simulink model "ifo_ut"  (Simulink 8.1)
settings: Solver=FixedStepDiscrete  StartTime=0.0  StopTime=10.0  FixedStep=0.005  RelTol=1e-3
PostLoadFcn:
  | , if any(exist('dsrtsu_mdlpostloadfcn', 'file') == [2, 3, 6]), try dsrtsu_mdlpostloadfcn('Execute', bdroot); catch fprintf('Error in PostLoadFcn (dsrtsu_mdlpostloadfcn) for model "%s":\n %s\n', bdroot, lasterr); end, end,
undefined symbols (not defined in the file or in its folder): VACC_ACCActing_flg, VACC_ACCOverride_flg, VACC_ACCRawTorqueReq_Nm, VACC_ACCSystemState_enum, VACC_DesiredDistance_m, VACC_StandstillClearance_m, VAEB_AEBActing_flg, VAEB_AEBSystemState_enum, VDHP_DisableACC_flg, VDHP_DisableADASFun_flg, VIFO_ACCCancelReq_flg, VIFO_ACCDist_flg, VIFO_ACCResSpdInc_flg, VIFO_ACCSetSpdDec_flg, VIFO_ACCTargetVehAssigned_flg, VIFO_ACCTargetVehRelSpeedX_mps, VIFO_ACCVehClearance_m, VIFO_DriverOvertakeReq_flg, VIFO_DriverSafetyStatusOk_flg, VIFO_DriverTurnSignalOn_flg, VIFO_VehicleStatusOk_flg, VPER_CameraStatus_enum, VPER_FusionStatus_enum, VPER_RadarStatus_enum
libraries: siltestlib x32, ifo x1
settings Model: DSRTSU_INTERNAL_RTI_VER=450  DSRTSU_INTERNAL_RTI_TYPE=rti1401  RTICANMMDATA=struct('GeneralSetupData',struct('modelroot','D:\ELN150201_TAIWAN\trunk\AdasDragon\software\sw_development\arch\app\ifo','generalsettings',struct('filesettings',struct('destfolder',struct('Name','RTICANMM_FILES','Check',1),'buildfolder',struct('Name','.','Check',1),'AbsDestfolder',struct('Name','D:\ELN150201_TAIWAN\trunk\AdasDragon\software\sw_development\arch\app\ifo\RTICANMM_FILES'),'AbsBuildfolder',struct('Name','D:\ELN150201_TAIWAN\trunk\AdasDragon\software\sw_development\arch\app\ifo'))),'options',struct('addpaths',1,'rmpaths',1,'addtrcexclusion',logical(1),'cannavigator',struct('checkmonitoring',0),'show_usrtrc',0,'use_usrtrc',0),'advanced',struct('options',[1 1 1 1 1 1 1 1 1 1 1 1 1 1 1 1 1 1 1 1 1 1 1 1 1 1 1 1 1 1 1 1 1 1 1 1 1 1 1 1 1 1 1 1 1 1 1 1 1 1 1 1 1 1 1 1 1 1 1 1 1 1 1 1 1 1 1 1 1 1 1 1 1 1 1 1 1 1 1 1 1 1 1 1 1 1 1 1 1 1 1 1 1 1 1 1 1 1 1 1]),'MPSetup',{{}},'modelname','ifo_ut','block','ifo_ut'))  DSRTSU_INTERNAL_RTIFPGA=40  Creator=xsellart  LastModifiedBy=AT015555
settings DataIOCC: SignalLoggingSaveFormat=Dataset
settings OptimizationCC: ExpressionDepthLimit=128
settings DebuggingCC: FcnCallInpInsideContextMsg=EnableAllAsError
settings HardwareCC: ProdIntDivRoundTo=Zero  ProdEndianess=BigEndian  ProdHWDeviceType=Generic->Custom  TargetIntDivRoundTo=Zero  TargetEndianess=BigEndian  TargetHWDeviceType=Generic->Custom
settings RTWCC: SystemTargetFile=rti1401.tlc  MakeCommand=make_rti  TemplateMakefile=rti1401.tmf  Description=dSPACE DS1401 Hardware Platform  ProcessScript=rti1401_make_rtw_hook
settings STFCustomTargetCC: CodeReplacementLibrary=ANSI_C  ParMdlRefBuildCompliant=on  GeneratePreprocessorConditionals=Disable all  SystemTargetFile=rti1401.tlc
settings GRTTargetCC: CompOptLevelCompliant=off  ConcurrentExecutionCompliant=off  MatFileLogging=off  ExtModeMexFile=noextcomm
settings CustomProperty: DataType=RTWOptions_EnumType_C__Program Files (x86)_dSPACE RCPHIL 2014-B_MATLAB_RTI_RTI1401_TLC_rti1401_1InitialSimState  Value=RUN
settings EnumStrPairs: String=RUN

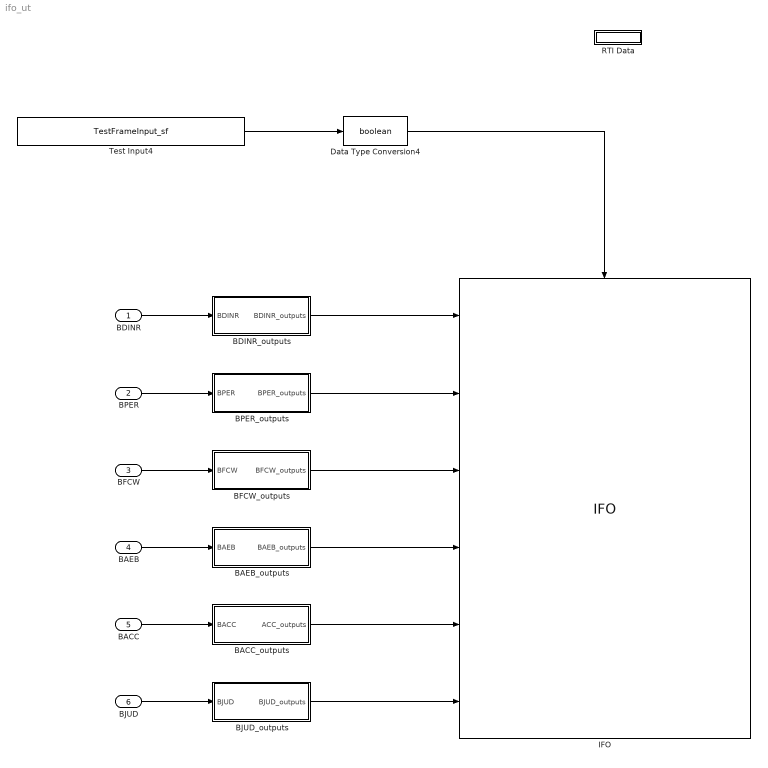
== system ifo_ut ==
  BDINR : Inport  OutDataTypeStr=Bus: BDINR_outputs
  BPER : Inport  Port=2  OutDataTypeStr=Bus: BPER_outputs
  BFCW : Inport  Port=3  OutDataTypeStr=Bus: BFCW_outputs
  BAEB : Inport  Port=4  OutDataTypeStr=Bus: BAEB_outputs
  BACC : Inport  Port=5  OutDataTypeStr=Bus: BACC_outputs
  BJUD : Inport  Port=6  OutDataTypeStr=Bus: BJUD_outputs
  BACC_outputs : Subsystem
  BAEB_outputs : Subsystem
  BDINR_outputs : Subsystem
  BFCW_outputs : Subsystem
  BJUD_outputs : Subsystem
  BPER_outputs : Subsystem
  Data Type Conversion4 : DataTypeConversion  OutDataTypeStr=boolean
  IFO : ifo/IFO
  RTI Data : Subsystem  Tag=struct('RTIDataServer',struct('RTIDataServerVs','2','RTIModelDescription','struct(''main'',''ifo_ut'',''sub'','''',''isMp'',0)'))  LoadFcn="if exist('rtidc'), try,  rtidc('DataHostBlockClbLoad', gcbh); catch, disp(['Warning: ''LoadFcn'' for RTI Data block failed: ' lasterr]); end, end,"  mask(RTI_DATA_HOST){}
      mask help:
      | RTI Data Block.
      | This block is used by RTI to store internal model-dependent data.
      | Please keep this block on the root level of the model. Deleting this block will result in data loss.
      |
      | NEVER DELETE OR COPY THIS BLOCK!
      settings: CopyFcn="if exist('rtidc'), try,  rtidc('DataHostBlockClbCopy', gcbh); catch, disp(['Warning: ''CopyFcn'' for RTI Data block failed: ' lasterr]); end, end,"  DeleteFcn="if exist('rtidc'), try,  rtidc('DataHostBlockClbDelete', gcbh); catch, disp(['Warning: ''DeleteFcn'' for RTI Data block failed: ' lasterr]); end, end,"  ModelCloseFcn="if exist('rtidc'), try,  rtidc('DataHostBlockClbModelClose', gcbh); catch, disp(['Warning: ''ModelCloseFcn'' for RTI Data block failed: ' lasterr]); end, end,"  PreSaveFcn="if exist('rtidc'), try,  rtidc('DataHostBlockClbPreSave', gcbh); catch, disp(['Warning: ''PreSaveFcn'' for RTI Data block failed: ' lasterr]); end, end,"  PostSaveFcn="if exist('rtidc'), try,  rtidc('DataHostBlockClbPostSave', gcbh); catch, disp(['Warning: ''PostSaveFcn'' for RTI Data block failed: ' lasterr]); end, end,"  NameChangeFcn="if exist('rtidc'), try,  rtidc('DataHostBlockClbNameChange', gcbh); catch, disp(['Warning: ''NameChangeFcn'' for RTI Data block failed: ' lasterr]); end, end,"
      mask Help:
      | RTI Data Block.
      | This block is used by RTI to store internal model-dependent data.
      | Please keep this block on the root level of the model. Deleting this block will result in data loss.
      | 
      | NEVER DELETE OR COPY THIS BLOCK!
      mask Display:
      | text(0.5, 0.5, 'RTI Data', 'HorizontalAlignment', 'center');
      | plot([1 0]);
  Test Input4 : S-Function  FunctionName=TestFrameInput_sf  Parameters=varname,sampletime  EnableBusSupport=off  mask(Test Input){varname=Scheduler_Trigger, sampletime=-1}
      mask prompts: varname "Name:"; sampletime "Sample Time:"
      mask help: Outputs the value of a Test Input variable from an Excel spreadsheet when used with the runsiltest script. Otherwise outputs 0.
      mask Display: fprintf('Test Input:\n%s',varname);
  wires:
  BDINR/1 -> BDINR_outputs/1(BDINR)
  BPER/1 -> BPER_outputs/1(BPER)
  BFCW/1 -> BFCW_outputs/1(BFCW)
  BJUD/1 -> BJUD_outputs/1(BJUD)
  BAEB/1 -> BAEB_outputs/1(BAEB)
  BACC/1 -> BACC_outputs/1(BACC)
  BFCW_outputs/1(BFCW_outputs) -> IFO/3
  BJUD_outputs/1(BJUD_outputs) -> IFO/6
  BACC_outputs/1(ACC_outputs) -> IFO/5
  BPER_outputs/1(BPER_outputs) -> IFO/2
  BDINR_outputs/1(BDINR_outputs) -> IFO/1
  BAEB_outputs/1(BAEB_outputs) -> IFO/4
  Test Input4/1 -> Data Type Conversion4/1
  Data Type Conversion4/1 -> IFO/Trigger

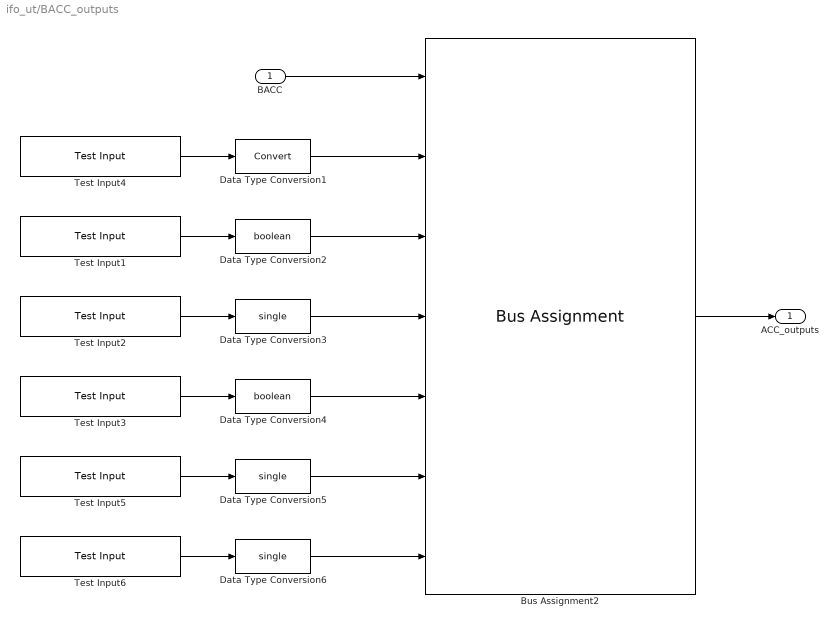
== system ifo_ut/BACC_outputs ==
  BACC : Inport  OutDataTypeStr=Bus: BACC_outputs
  Bus Assignment2 : BusAssignment  AssignedSignals=VACC_ACCSystemState_enum,VACC_ACCActing_flg,VACC_ACCRawTorqueReq_Nm,VACC_ACCOverride_flg,VACC_DesiredDistance_m,VACC_StandstillClearance_m
  Data Type Conversion1 : DataTypeConversion
  Data Type Conversion2 : DataTypeConversion  OutDataTypeStr=boolean
  Data Type Conversion3 : DataTypeConversion  OutDataTypeStr=single
  Data Type Conversion4 : DataTypeConversion  OutDataTypeStr=boolean
  Data Type Conversion5 : DataTypeConversion  OutDataTypeStr=single
  Data Type Conversion6 : DataTypeConversion  OutDataTypeStr=single
  Test Input1 : siltestlib/Test Input  varname=VACC_ACCActing_flg  sampletime=-1
  Test Input2 : siltestlib/Test Input  varname=VACC_ACCRawTorqueReq_Nm  sampletime=-1
  Test Input3 : siltestlib/Test Input  varname=VACC_ACCOverride_flg  sampletime=-1
  Test Input4 : siltestlib/Test Input  varname=VACC_ACCSystemState_enum  sampletime=-1
  Test Input5 : siltestlib/Test Input  varname=VACC_DesiredDistance_m  sampletime=-1
  Test Input6 : siltestlib/Test Input  varname=VACC_StandstillClearance_m  sampletime=-1
  ACC_outputs : Outport  OutDataTypeStr=Bus: BAEB_outputs
  wires:
  Test Input4/1 -> Data Type Conversion1/1
  Bus Assignment2/1 -> ACC_outputs/1
  BACC/1 -> Bus Assignment2/1
  Test Input1/1 -> Data Type Conversion2/1
  Test Input2/1 -> Data Type Conversion3/1
  Test Input3/1 -> Data Type Conversion4/1
  Test Input5/1 -> Data Type Conversion5/1
  Test Input6/1 -> Data Type Conversion6/1
  Data Type Conversion1/1 -> Bus Assignment2/2
  Data Type Conversion6/1 -> Bus Assignment2/7
  Data Type Conversion2/1 -> Bus Assignment2/3
  Data Type Conversion5/1 -> Bus Assignment2/6
  Data Type Conversion4/1 -> Bus Assignment2/5
  Data Type Conversion3/1 -> Bus Assignment2/4

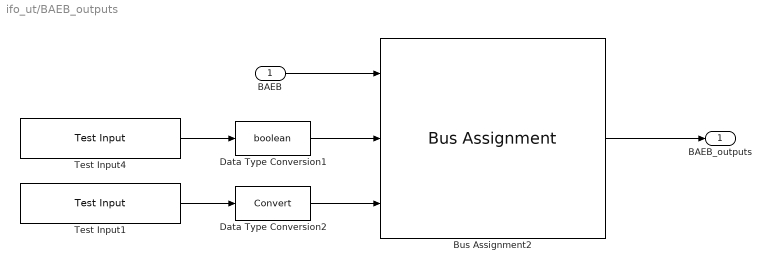
== system ifo_ut/BAEB_outputs ==
  BAEB : Inport  OutDataTypeStr=Bus: BAEB_outputs
  Bus Assignment2 : BusAssignment  AssignedSignals=VAEB_AEBActing_flg,VAEB_AEBSystemState_enum
  Data Type Conversion1 : DataTypeConversion  OutDataTypeStr=boolean
  Data Type Conversion2 : DataTypeConversion
  Test Input1 : siltestlib/Test Input  varname=VAEB_AEBSystemState_enum  sampletime=-1
  Test Input4 : siltestlib/Test Input  varname=VAEB_AEBActing_flg  sampletime=-1
  BAEB_outputs : Outport  OutDataTypeStr=Bus: BAEB_outputs
  wires:
  BAEB/1 -> Bus Assignment2/1
  Bus Assignment2/1 -> BAEB_outputs/1
  Test Input4/1 -> Data Type Conversion1/1
  Data Type Conversion1/1 -> Bus Assignment2/2
  Test Input1/1 -> Data Type Conversion2/1
  Data Type Conversion2/1 -> Bus Assignment2/3

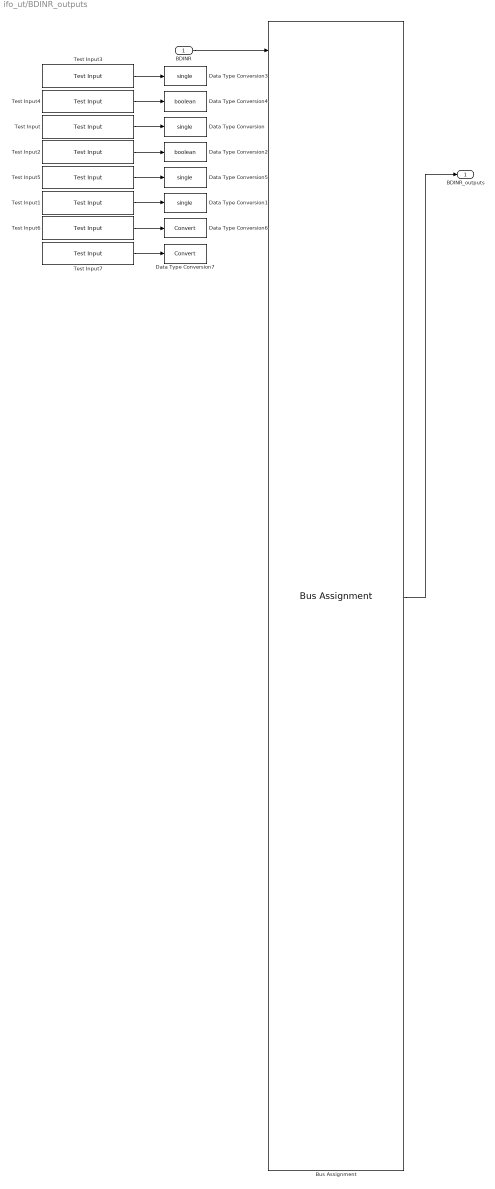
== system ifo_ut/BDINR_outputs ==
  BDINR : Inport  OutDataTypeStr=Bus: BDINR_outputs
  Bus Assignment : BusAssignment  AssignedSignals=VDINR_VehSpd_mps,VDINR_YawRate_degps,VDINR_SeatBeltNOTFasten_flg,VDINR_VehCrashed_flg,VDINR_TCSActive_flg,VDINR_VehSpdValid_flg,VDINR_LongAccelValid_flg,VDINR_LatAccelValid_flg,VDINR_YawRateValid_flg,VDINR_SteerAngleValid_flg,VDINR_SteerSpeedValid_flg,VDINR_HWAccelPedalPosnValid_flg,VDINR_DriverBrakPedalOnValid_flg,VDINR_NowGearPosnValid_flg,VDINR_ESCFault_flg,VDINR_ABSFault_flg,VDINR_EMSOpState_enum,VDINR_EPASMILReq_flg,VDINR_TCMFaultStatus_enum,VDINR_DriverDoorOpen_flg,VDINR_PassengerDoorOpen_flg,VDINR_LRDoorOpen_flg,VDINR_RRDoorOpen_flg,VDINR_SteerSpeed_degps,VDINR_SteerAngle_deg,VDINR_HWAccelPedalPosn_pct,VDINR_ParkBrakeBindSta_enum,VDINR_MCPressure_bar,VDINR_DriverBrakPedalOn_flg,VDINR_NowGearPosn_enum,VDINR_ACCOnVCU_flg,VDINR_TurnSignalSwL_flg,VDINR_TurnSignalSwR_flg,VDINR_LongAccel_G,VDINR_ACCSetSpdDecH_flg,VDINR_ACCSpdDecH_flg,VDINR_ACCResSpdIncH_flg,VDINR_ACCSpdIncH_flg,VDINR_ACCSetSpdDecVCU_flg,VDINR_ACCResSpdIncVCU_flg,VDINR_ACCDistVCU_flg,VDINR_ACCTimeGapDecH_flg,VDINR_ACCOnH_flg
  Data Type Conversion{,1,3,5} (4 alike) : DataTypeConversion  OutDataTypeStr=single
  Data Type Conversion2 : DataTypeConversion  OutDataTypeStr=boolean
  Data Type Conversion4 : DataTypeConversion  OutDataTypeStr=boolean
  Data Type Conversion6 : DataTypeConversion
  Data Type Conversion7 : DataTypeConversion
  Test Input : siltestlib/Test Input  varname=VDINR_VehSpd_kph  sampletime=-1
  Test Input1 : siltestlib/Test Input  varname=VDINR_CurDriverTqReq_Nm  sampletime=-1
  Test Input2 : siltestlib/Test Input  varname=VDINR_DriverBrakPedalOn_flg  sampletime=-1
  Test Input3 : siltestlib/Test Input  varname=VDINR_VehSpd_mps  sampletime=-1
  Test Input4 : siltestlib/Test Input  varname=VDINR_HMICANValid_flg  sampletime=-1
  Test Input5 : siltestlib/Test Input  varname=VDINR_HWAccelPedalPosn_pct  sampletime=-1
  Test Input6 : siltestlib/Test Input  varname=VDINR_NowGearPosn_enum  sampletime=-1
  Test Input7 : siltestlib/Test Input  varname=VDINR_ParkBrakeBindSta_enum  sampletime=-1
  BDINR_outputs : Outport  OutDataTypeStr=Bus: BDINR_outputs
  wires:
  Bus Assignment/1 -> BDINR_outputs/1
  BDINR/1 -> Bus Assignment/1
  Test Input/1 -> Data Type Conversion/1
  Test Input1/1 -> Data Type Conversion1/1
  Test Input2/1 -> Data Type Conversion2/1
  Test Input3/1 -> Data Type Conversion3/1
  Test Input4/1 -> Data Type Conversion4/1
  Test Input5/1 -> Data Type Conversion5/1
  Test Input6/1 -> Data Type Conversion6/1
  Test Input7/1 -> Data Type Conversion7/1

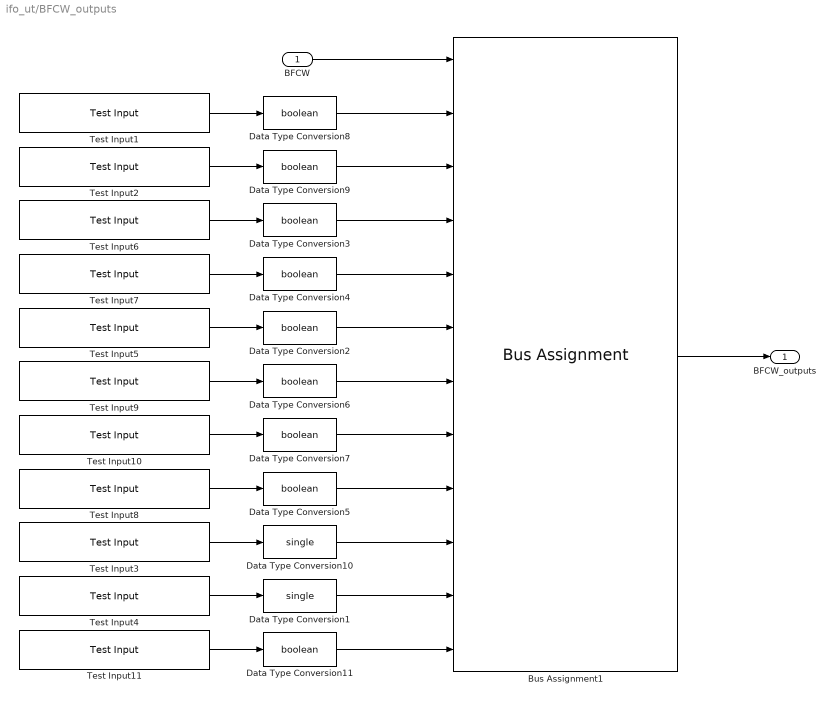
== system ifo_ut/BFCW_outputs ==
  BFCW : Inport  OutDataTypeStr=Bus: BFCW_outputs
  Bus Assignment1 : BusAssignment  AssignedSignals=VIFO_ACCSetSpdDec_flg,VIFO_ACCResSpdInc_flg,VIFO_ACCDist_flg,VIFO_ACCCancelReq_flg,VIFO_DriverOvertakeReq_flg,VIFO_VehicleStatusOk_flg,VIFO_DriverSafetyStatusOk_flg,VIFO_ACCTargetVehAssigned_flg,VIFO_ACCTargetVehRelSpeedX_mps,VIFO_ACCVehClearance_m,VIFO_DriverTurnSignalOn_flg
  Data Type Conversion1 : DataTypeConversion  OutDataTypeStr=single
  Data Type Conversion10 : DataTypeConversion  OutDataTypeStr=single
  Data Type Conversion{2..9,11} (9 alike) : DataTypeConversion  OutDataTypeStr=boolean
  Test Input1 : siltestlib/Test Input  varname=VIFO_ACCSetSpdDec_flg  sampletime=-1
  Test Input10 : siltestlib/Test Input  varname=VIFO_DriverSafetyStatusOk_flg  sampletime=-1
  Test Input11 : siltestlib/Test Input  varname=VIFO_DriverTurnSignalOn_flg  sampletime=-1
  Test Input2 : siltestlib/Test Input  varname=VIFO_ACCResSpdInc_flg  sampletime=-1
  Test Input3 : siltestlib/Test Input  varname=VIFO_ACCTargetVehRelSpeedX_mps  sampletime=-1
  Test Input4 : siltestlib/Test Input  varname=VIFO_ACCVehClearance_m  sampletime=-1
  Test Input5 : siltestlib/Test Input  varname=VIFO_DriverOvertakeReq_flg  sampletime=-1
  Test Input6 : siltestlib/Test Input  varname=VIFO_ACCDist_flg  sampletime=-1
  Test Input7 : siltestlib/Test Input  varname=VIFO_ACCCancelReq_flg  sampletime=-1
  Test Input8 : siltestlib/Test Input  varname=VIFO_ACCTargetVehAssigned_flg  sampletime=-1
  Test Input9 : siltestlib/Test Input  varname=VIFO_VehicleStatusOk_flg  sampletime=-1
  BFCW_outputs : Outport  OutDataTypeStr=Bus: BFCW_outputs
  wires:
  BFCW/1 -> Bus Assignment1/1
  Bus Assignment1/1 -> BFCW_outputs/1
  Test Input1/1 -> Data Type Conversion8/1
  Data Type Conversion8/1 -> Bus Assignment1/2
  Test Input2/1 -> Data Type Conversion9/1
  Data Type Conversion9/1 -> Bus Assignment1/3
  Test Input3/1 -> Data Type Conversion10/1
  Data Type Conversion3/1 -> Bus Assignment1/4
  Test Input4/1 -> Data Type Conversion1/1
  Data Type Conversion1/1 -> Bus Assignment1/11
  Data Type Conversion10/1 -> Bus Assignment1/10
  Test Input5/1 -> Data Type Conversion2/1
  Data Type Conversion2/1 -> Bus Assignment1/6
  Test Input6/1 -> Data Type Conversion3/1
  Data Type Conversion4/1 -> Bus Assignment1/5
  Test Input7/1 -> Data Type Conversion4/1
  Data Type Conversion5/1 -> Bus Assignment1/9
  Test Input8/1 -> Data Type Conversion5/1
  Data Type Conversion6/1 -> Bus Assignment1/7
  Test Input9/1 -> Data Type Conversion6/1
  Data Type Conversion7/1 -> Bus Assignment1/8
  Test Input10/1 -> Data Type Conversion7/1
  Test Input11/1 -> Data Type Conversion11/1
  Data Type Conversion11/1 -> Bus Assignment1/12

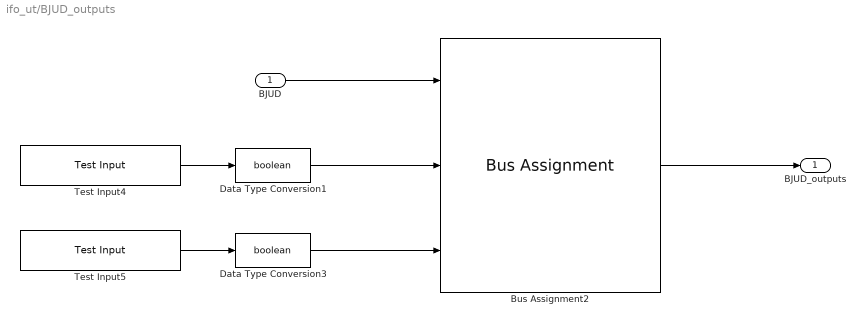
== system ifo_ut/BJUD_outputs ==
  BJUD : Inport  OutDataTypeStr=Bus: BJUD_outputs
  Bus Assignment2 : BusAssignment  AssignedSignals=VDHP_DisableADASFun_flg,VDHP_DisableACC_flg
  Data Type Conversion1 : DataTypeConversion  OutDataTypeStr=boolean
  Data Type Conversion3 : DataTypeConversion  OutDataTypeStr=boolean
  Test Input4 : siltestlib/Test Input  varname=VDHP_DisableADASFun_flg  sampletime=-1
  Test Input5 : siltestlib/Test Input  varname=VDHP_DisableACC_flg  sampletime=-1
  BJUD_outputs : Outport  OutDataTypeStr=Bus: BJUD_outputs
  wires:
  BJUD/1 -> Bus Assignment2/1
  Bus Assignment2/1 -> BJUD_outputs/1
  Test Input4/1 -> Data Type Conversion1/1
  Data Type Conversion1/1 -> Bus Assignment2/2
  Test Input5/1 -> Data Type Conversion3/1
  Data Type Conversion3/1 -> Bus Assignment2/3

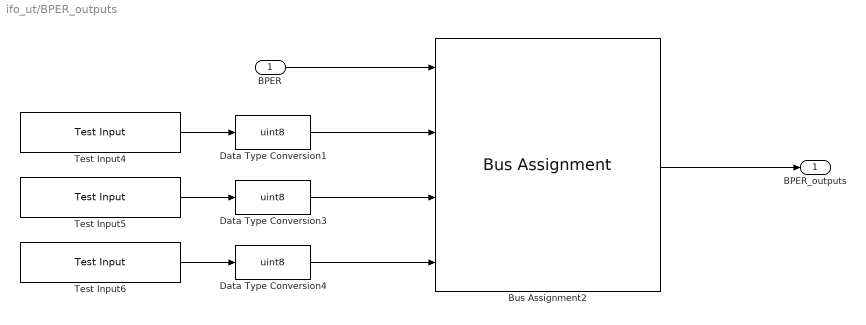
== system ifo_ut/BPER_outputs ==
  BPER : Inport  OutDataTypeStr=Bus: BPER_outputs
  Bus Assignment2 : BusAssignment  AssignedSignals=VPER_CameraStatus_enum,VPER_RadarStatus_enum,VPER_FusionStatus_enum
  Data Type Conversion1 : DataTypeConversion  OutDataTypeStr=uint8
  Data Type Conversion3 : DataTypeConversion  OutDataTypeStr=uint8
  Data Type Conversion4 : DataTypeConversion  OutDataTypeStr=uint8
  Test Input4 : siltestlib/Test Input  varname=VPER_CameraStatus_enum  sampletime=-1
  Test Input5 : siltestlib/Test Input  varname=VPER_RadarStatus_enum  sampletime=-1
  Test Input6 : siltestlib/Test Input  varname=VPER_FusionStatus_enum  sampletime=-1
  BPER_outputs : Outport  OutDataTypeStr=Bus: BPER_outputs
  wires:
  BPER/1 -> Bus Assignment2/1
  Bus Assignment2/1 -> BPER_outputs/1
  Test Input4/1 -> Data Type Conversion1/1
  Data Type Conversion1/1 -> Bus Assignment2/2
  Test Input5/1 -> Data Type Conversion3/1
  Data Type Conversion3/1 -> Bus Assignment2/3
  Test Input6/1 -> Data Type Conversion4/1
  Data Type Conversion4/1 -> Bus Assignment2/4

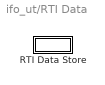
== system ifo_ut/RTI Data ==
  RTI Data Store : Subsystem  Tag=struct('private',struct('version',struct('dsVer',uint32(2),'dsVerCreation',uint32(2),'RTI',struct('ver','7.3','type','RTI1401')),'access',struct('type','Model','isPerm',1,'created',['29-Oct-2015 16:31:40'],'modified',['10-Apr-2017 10:25:40'],'location','')),'public',struct('main',struct('data',[]),'sub',struct('name','','data',[])))  mask(RTI_DATA_STORE){}
      mask help:
      | RTI Data Store Block. This block is used by RTI to store internal model dependent data. Deleting this block will result in data loss.
      |
      | NEVER DELETE, COPY, OR MODIFY THIS BLOCK!
      mask Help:
      | RTI Data Store Block. This block is used by RTI to store internal model dependent data. Deleting this block will result in data loss.
      | 
      | NEVER DELETE, COPY, OR MODIFY THIS BLOCK!
      mask Display: text(0.5, 0.5, ' ', 'HorizontalAlignment', 'center');

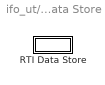
== system ifo_ut/RTI Data/RTI Data Store ==
  RTI Data Store : Subsystem  mask(RTI_DATA_STORE){}
      mask help:
      | RTI Data Store Block. This block is used by RTI to store internal model dependent data. Deleting this block will result in data loss.
      |
      | NEVER DELETE, COPY, OR MODIFY THIS BLOCK!
      mask Help:
      | RTI Data Store Block. This block is used by RTI to store internal model dependent data. Deleting this block will result in data loss.
      | 
      | NEVER DELETE, COPY, OR MODIFY THIS BLOCK!
      mask Display: text(0.5, 0.5, ' ', 'HorizontalAlignment', 'center');

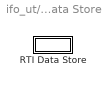
== system ifo_ut/RTI Data/RTI Data Store/RTI Data Store ==
  RTI Data Store : Subsystem  mask(RTI_DATA_STORE){}
      mask help:
      | RTI Data Store Block. This block is used by RTI to store internal model dependent data. Deleting this block will result in data loss.
      |
      | NEVER DELETE, COPY, OR MODIFY THIS BLOCK!
      mask Help:
      | RTI Data Store Block. This block is used by RTI to store internal model dependent data. Deleting this block will result in data loss.
      | 
      | NEVER DELETE, COPY, OR MODIFY THIS BLOCK!
      mask Display: text(0.5, 0.5, ' ', 'HorizontalAlignment', 'center');

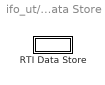
== system ifo_ut/RTI Data/RTI Data Store/RTI Data Store/RTI Data Store ==
  RTI Data Store : Subsystem  mask(RTI_DATA_STORE){}
      mask help:
      | RTI Data Store Block. This block is used by RTI to store internal model dependent data. Deleting this block will result in data loss.
      |
      | NEVER DELETE, COPY, OR MODIFY THIS BLOCK!
      mask Help:
      | RTI Data Store Block. This block is used by RTI to store internal model dependent data. Deleting this block will result in data loss.
      | 
      | NEVER DELETE, COPY, OR MODIFY THIS BLOCK!
      mask Display: text(0.5, 0.5, ' ', 'HorizontalAlignment', 'center');

== system ifo_ut/RTI Data/RTI Data Store/RTI Data Store/RTI Data Store/RTI Data Store ==
